simulink model "modelWithSimplifiedSystemDynamics"  (R2020b)
settings: Solver=VariableStepAuto  StartTime=0.0  StopTime=20  MaxStep=0.1  RelTol=1e-2  AbsTol=1e-2
undefined symbols (not defined in the file): configSequence
libraries: robotmaniplib x1, robotcorelib x1
settings Model: PauseTimes=3.1  OrderedModelArguments=off  Creator=The MathWorks, Inc.  LastModifiedBy=shuali

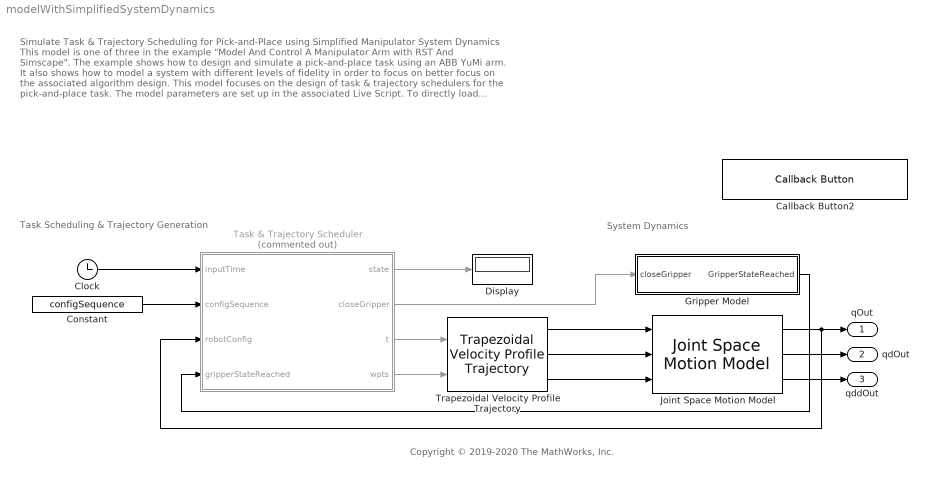
== system modelWithSimplifiedSystemDynamics ==
  note: Task Scheduling & Trajectory Generation
  note: System Dynamics
  note: Copyright © 2019-2020 The MathWorks, Inc.
  note: Simulate Task & Trajectory Scheduling for Pick-and-Place using Simplified Manipulator System Dynamics
      | This model is one of three in the example "Model And Control A Manipulator Arm with RST And Simscape". The example shows how to design and simulate a pick-and-place task using an ABB YuMi arm. It also shows how to model a system with different levels of fidelity in order to focus on better focus on the associated algorithm design. This model focuses on the design of task & trajectory schedulers for the pick-and-place task.
      |
      | The model parameters are set up in the associated Live Script. To directly load default parameters and run the model, click the "Load Default Parameters" button and simulate. Please be aware that this will overwrite any existing variables in the MATLAB workspace.
  Callback Button2 : CallbackButton  ButtonText=Load Default Parameters (will overwrite workspace)
      settings: ClickFcn=|
      | robot = loadrobot('abbYumi', 'Gravity', [0 0 -9.81]);
      | load abbExampleRSTVariables.mat;
  Clock : Clock
  Constant : Constant  Value=configSequence
  Display : Display
  Gripper Model : Subsystem
  Joint Space Motion Model : robotmaniplib/Joint Space Motion Model  RigidBodyTree=robot  MotionType=Independent Joint Motion  ProportionalGain=100  DerivativeGain=10  ErrorDynamicsSpecification=Damping Ratio / Natural Frequency  DampingRatio=1  NaturalFrequency=10  SettlingTime=0.59  Overshoot=0  ShowExternalForcePort=off  InitConfig=q0  InitJointVel=dq0  SimulateUsing=Interpreted execution
      settings: SourceProductName=Robotics System Toolbox
  Task & Trajectory Scheduler : MATLAB Function  Commented=on  TreatAsAtomicUnit=on
  Trapezoidal Velocity Profile Trajectory : robotcorelib/Trapezoidal Velocity Profile Trajectory  WaypointSource=External  Waypoints=[ 0, -0.5, -1; 0, 0.5, 1 ]  NumParams=1  Parameter1=End Time  Parameter2=End Time  ParameterSource=Internal  PeakVelocity=[ 2; 2 ]  Acceleration=[ 1; 2 ]  EndTime=2  AccelTime=[ 1; 2 ]  SimulateUsing=Interpreted execution
      settings: SourceProductName=Robotics System Toolbox
  qOut : Outport
  qdOut : Outport  Port=2
  qddOut : Outport  Port=3
  wires:
  Task & Trajectory Scheduler/3(t) -> Trapezoidal Velocity Profile Trajectory/1
  Task & Trajectory Scheduler/4(wpts) -> Trapezoidal Velocity Profile Trajectory/2
  Constant/1 -> Task & Trajectory Scheduler/2(configSequence)
  Task & Trajectory Scheduler/1(state) -> Display/1
  Clock/1 -> Task & Trajectory Scheduler/1(inputTime)
  Joint Space Motion Model/2 -> qdOut/1
  Joint Space Motion Model/3 -> qddOut/1
  Joint Space Motion Model/1 -> Task & Trajectory Scheduler/3(robotConfig), qOut/1
  Trapezoidal Velocity Profile Trajectory/3 -> Joint Space Motion Model/3
  Trapezoidal Velocity Profile Trajectory/2 -> Joint Space Motion Model/2
  Trapezoidal Velocity Profile Trajectory/1 -> Joint Space Motion Model/1
  Task & Trajectory Scheduler/2(closeGripper) -> Gripper Model/1(closeGripper)
  Gripper Model/1(GripperStateReached) -> Task & Trajectory Scheduler/4(gripperStateReached)

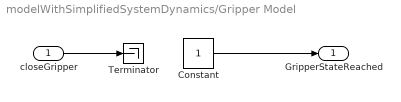
== system modelWithSimplifiedSystemDynamics/Gripper Model ==
  closeGripper : Inport
  Constant : Constant
  Terminator : Terminator
  GripperStateReached : Outport
  wires:
  Constant/1 -> GripperStateReached/1
  closeGripper/1 -> Terminator/1

== matlab function modelWithSimplifiedSystemDynamics/Task & Trajectory Scheduler ==
  settings: updateMethod=DISCRETE
  data: inputTime input; configSequence input; state output; closeGripper output; robotConfig input; t output; wpts output; gripperStateReached input
function [state, closeGripper, t, wpts] = commandLogic(inputTime, configSequence, robotConfig, gripperStateReached)

persistent motionState
persistent resetTimeValue

% Set some variables
posTgtThreshold = 0.015;

% Initialize persistent variables
if isempty(motionState)
    motionState = 0;
end
if isempty(resetTimeValue)
    resetTimeValue = 0;
end

% Output the state and time
state = motionState;
t = inputTime - resetTimeValue;

% Initialize outputs to starting state
wpts = configSequence(:,1:2);
closeGripper = false;

switch motionState
    case 1
        % Grasp: Move from approach to grasp & open the gripper
        wpts = configSequence(:,2:3);
        closeGripper = false;
    case 2
        % Close the gripper
        wpts = [configSequence(:,3) configSequence(:,3)];
        closeGripper = true;
    case 3
        % Depart grasp
        wpts = configSequence(:,3:4);
        closeGripper = true;
    case 4
        % Move to place approach
        wpts = configSequence(:,4:5);
        closeGripper = true;
    case 5
        % Move to place
        wpts = configSequence(:,5:6);
        closeGripper = true;
    case 6
        % Open the gripper
        wpts = [configSequence(:,6) configSequence(:,6)];
        closeGripper = false;
    case 7
        % Depart place
        wpts = configSequence(:,6:7);
        closeGripper = false;
    case 8
        % Cycle to grasp approach
        wpts = configSequence(:,[7 2]);
        closeGripper = false;
end
   
% Get the current status
trajEndConfigReached = endStateReached(robotConfig, wpts, posTgtThreshold);

% Advance the state and reset time as needed
if trajEndConfigReached && gripperStateReached
    % Advance the state and reset the time
    motionState = mod(motionState, 7) + 1;
    resetTimeValue = inputTime;
end

end

function isReached = endStateReached(config, wpts, tgtThreshold)
    
    % Initialize output
    isReached = false;
    
    % Mark config states that are specific to gripper
    armStateExclGripperIdx = 10:16;
    
    %Extract the arm that matters and then ignore the gripper position
    armConfig = config(armStateExclGripperIdx,:);
    armTarget = wpts(armStateExclGripperIdx,2);
    
    % Check if the arm states match the target waypoints
    diffWpts = zeros(length(armStateExclGripperIdx),1);
    diffWpts(:,:) = abs(armConfig - armTarget);
    errorStatus = diffWpts < tgtThreshold;
    if all(errorStatus)
        isReached = true;
    end
end
